simulink model "sm_control_feedforward_buck"  (R2016a)
settings: Solver=VariableStepAuto  StartTime=0.0  StopTime=5  RelTol=1e-3
libraries: powerlib x10, simulink x1
settings Model: Creator=jorda  LastModifiedBy=jorda

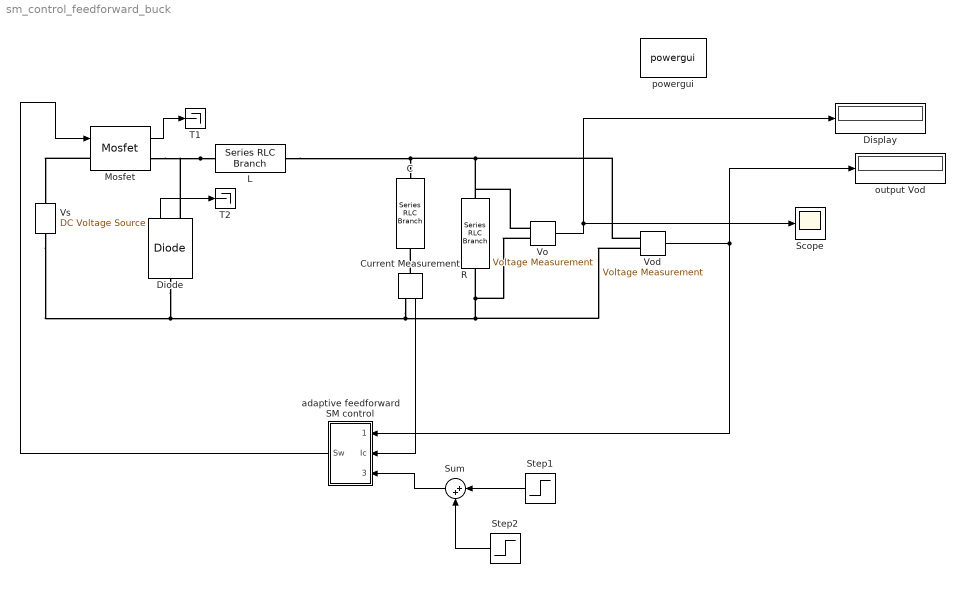
== system sm_control_feedforward_buck ==
  C : powerlib/Elements/Series RLC Branch  LConnTagsString=__new0  RConnTagsString=__new0  BranchType=C  Resistance=1  Inductance=1e-3  SetiL0=off  InitialCurrent=0  Capacitance=2000e-6  Setx0=off  InitialVoltage=0  Measurements=None
  Current Measurement : powerlib/Measurements/Current Measurement  PhasorSimulation=off  OutputType=Complex  PSBequivalent=0
  Diode : powerlib/Power Electronics/Diode  Ron=0.001  Lon=0  Vf=0.8  IC=0  UseSnubber=off  Rs=500  Cs=250e-9  Measurements=on
  Display : Display
  L : powerlib/Elements/Series RLC Branch  LConnTagsString=__new0  RConnTagsString=__new0  BranchType=L  Resistance=1  Inductance=2e-3  SetiL0=off  InitialCurrent=0  Capacitance=1e-6  Setx0=off  InitialVoltage=0  Measurements=None
  Mosfet : powerlib/Power Electronics/Mosfet  Ron=0.1  Lon=0  Rd=0.01  Vfd=0  IC=0  Rs=1e5  Cs=inf  Measurements=on
  R : powerlib/Elements/Series RLC Branch  LConnTagsString=__new0  RConnTagsString=__new0  BranchType=R  Resistance=4  Inductance=1e-3  SetiL0=off  InitialCurrent=0  Capacitance=1e-6  Setx0=off  InitialVoltage=0  Measurements=None
  Scope : Scope
  Step1 : Step  Before=4  After=5  SampleTime=0
  Step2 : Step  Time=3  After=-2  SampleTime=0
  Sum : Sum  Inputs=|++
  T1 : Terminator
  T2 : Terminator
  Vo : powerlib/Measurements/Voltage Measurement  PhasorSimulation=off  OutputType=Complex  PSBequivalent=0
  Vod : powerlib/Measurements/Voltage Measurement  PhasorSimulation=off  OutputType=Complex  PSBequivalent=0
  Vs : powerlib/Electrical Sources/DC Voltage Source  Amplitude=15  Measurements=None
  adaptive feedforward SM control : Subsystem
  output Vod : Display
  powergui : powerlib/powergui  Priority=1  SimulationMode=Continuous  SolverType=Tustin/Backward Euler (TBE)  SampleTime=50e-6  frequency=60  SPID=off  DisableSnubberDevices=off  DisableRonSwitches=off  DisableVfSwitches=off  SwTol=0  DisplayEquations=off  Interpol=off  ExternalGateDelay=off  methode=off  Ts=10  FunctionMessages=off  echomessages=off  HookPort=off  EnableUseOfTLC=off  x0status=blocks  frequencyindice=0  Pbase=100e6  ErrMax=1e-4  Iterations=50  UnitsV=kV  UnitsW=MW  buscounter=0  RestoreLinks=warning  ResistiveCurrentMeasurement=off  Frange=[0:2:500]  Ylog=off  Xlog=on  ShowGrid=off  save=off  variable=ZData  structure=0  ZoomFFT=off  StartTime=0.0  cycles=1  DisplayStyle=1  fundamental=60  FreqAxis=off  MaxFrequency=1000  frequencyindicesteady=1  RmsSteady=1  display=off
  wires:
  Diode/1 -> T2/1
  Mosfet/1 -> T1/1
  Current Measurement/1 -> adaptive feedforward SM control/2(Ic)
  adaptive feedforward SM control/1(Sw) -> Mosfet/1
  Vod/1 -> adaptive feedforward SM control/1(Vod), output Vod/1
  Vo/1 -> Scope/1, Display/1
  Step1/1 -> Sum/1
  Sum/1 -> adaptive feedforward SM control/3(Vref)
  Step2/1 -> Sum/2
  connections:
  L/RConn1 -- Vod/LConn1 -- R/LConn1 -- Vo/LConn1 -- C/LConn1
  Diode/LConn1 -- Vs/LConn1 -- Current Measurement/RConn1 -- Vod/LConn2 -- R/RConn1 -- Vo/LConn2
  L/LConn1 -- Mosfet/RConn1 -- Diode/RConn1
  Current Measurement/LConn1 -- C/RConn1
  Mosfet/LConn1 -- Vs/RConn1

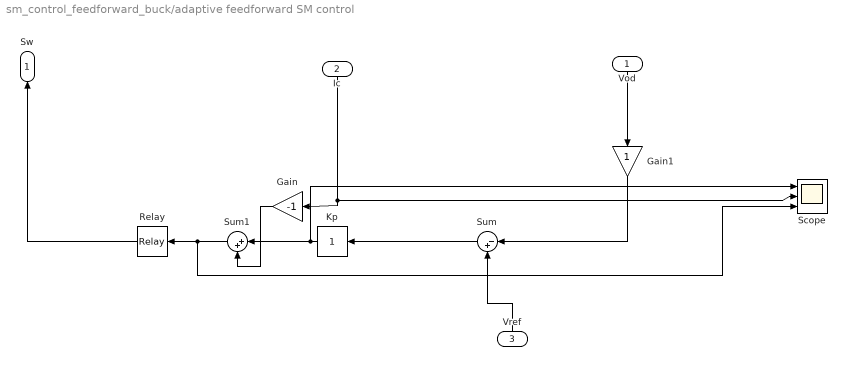
== system sm_control_feedforward_buck/adaptive feedforward SM control ==
  Vod : Inport
  Ic : Inport  Port=2
  Vref : Inport  Port=3
  Gain : Gain  Gain=-1  ParamDataTypeStr=double  OutDataTypeStr=double
  Gain1 : Gain  ParamDataTypeStr=double  OutDataTypeStr=double
  Kp : simulink/Math Operations/Slider Gain  low=0  gain=1  high=8000
  Relay : Relay  OnSwitchValue=0.79  OffSwitchValue=-0.79  OutDataTypeStr=Inherit: Inherit via back propagation
  Scope : Scope  NumInputPorts=3
  Sum : Sum  Inputs=|-+  AccumDataTypeStr=single  OutDataTypeStr=double  InputSameDT=on
  Sum1 : Sum  Inputs=|++  AccumDataTypeStr=double  OutDataTypeStr=double  InputSameDT=on
  Sw : Outport
  wires:
  Gain1/1 -> Sum/1
  Ic/1 -> Scope/2, Gain/1
  Vod/1 -> Gain1/1
  Sum1/1 -> Scope/3, Relay/1
  Kp/1 -> Sum1/1, Scope/1
  Sum/1 -> Kp/1
  Gain/1 -> Sum1/2
  Relay/1 -> Sw/1
  Vref/1 -> Sum/2
